simulink model "Regulation_tuning_2024b"  (R2024b)
settings: Solver=FixedStepAuto  StartTime=0.0  StopTime=10.0  FixedStep=0.001  RelTol=1e-3
values from neighbouring files (symbols this model uses):
  theta0 = -pi/2    (= -1.57079632679)    [automated_tuning_simulation.m]    (also in regulation_tuning_simulation.m = 0.785398163397; simulation.m = 0.785398163397; tuning_simulation.m = 0.785398163397)
  x0 = S.traj.xy(1,1)    [automated_tuning_simulation.m]    (also in regulation_tuning_simulation.m = -0.8; simulation.m; tuning_simulation.m)
  x_box = 850    [parking_box.mat]    (also in regulation_tuning_simulation.m = 0; replay_q_timeseries_on_maze_pacman.m; replay_q_timeseries_on_maze_pacman_real.m; simulation.m)
  y0 = S.traj.xy(1,2)    [automated_tuning_simulation.m]    (also in regulation_tuning_simulation.m = 0.5; simulation.m; tuning_simulation.m)
  y_box = 880    [parking_box.mat]    (also in regulation_tuning_simulation.m = 0; replay_q_timeseries_on_maze_pacman.m; replay_q_timeseries_on_maze_pacman_real.m; simulation.m)
undefined symbols (not defined in the file or in its folder): kd, kv, kw
settings Model: Creator=david  LastModifiedBy=emica
settings DataIOCC: ReturnWorkspaceOutputs=off

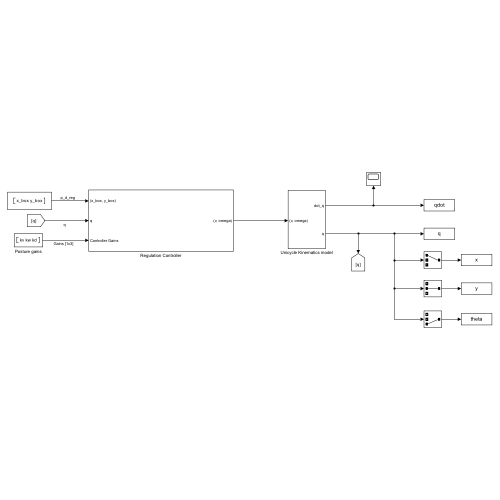
[thumbnail: Simulink's stored preview of the top-level diagram]
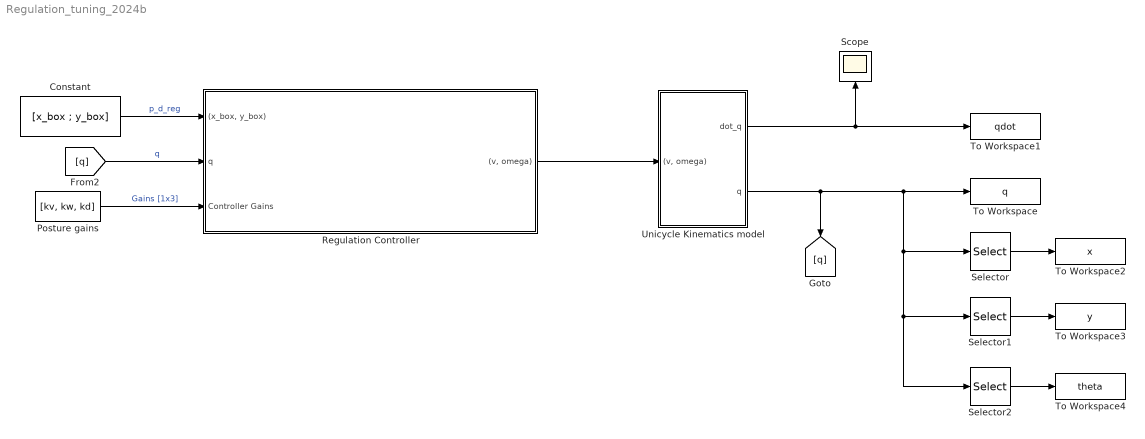
== system Regulation_tuning_2024b ==
  Constant : Constant  Value=[x_box ; y_box]
  Posture gains : Constant  Value=[kv, kw, kd]
  Regulation Controller : Subsystem
  Scope : Scope
  Selector : Selector  InputPortWidth=3  IndexOptions=Index vector (dialog)  Indices=[1]  OutputSizes=1
  Selector1 : Selector  InputPortWidth=3  IndexOptions=Index vector (dialog)  Indices=[2]  OutputSizes=1
  Selector2 : Selector  InputPortWidth=3  IndexOptions=Index vector (dialog)  Indices=[3]  OutputSizes=1
  To Workspace : ToWorkspace  VariableName=q  SaveFormat=Timeseries  SampleTime=-1
  To Workspace1 : ToWorkspace  VariableName=qdot  SaveFormat=Timeseries  SampleTime=-1
  To Workspace2 : ToWorkspace  VariableName=x  SaveFormat=Timeseries  SampleTime=-1
  To Workspace3 : ToWorkspace  VariableName=y  SaveFormat=Timeseries  SampleTime=-1
  To Workspace4 : ToWorkspace  VariableName=theta  SaveFormat=Timeseries  SampleTime=-1
  Unicycle Kinematics model : Subsystem
  wires:
  Regulation Controller/1("(v, omega)") -> Unicycle Kinematics model/1("(v, omega)")
  Constant/1 -> Regulation Controller/1("(x_box, y_box)")  "p_d_reg"
  Unicycle Kinematics model/1(dot_q) -> To Workspace1/1, Scope/1
  [q] -> Regulation Controller/2(q)  "q"
  Posture gains/1 -> Regulation Controller/3(Controller Gains)  "Gains [1x3]"
  Selector/1 -> To Workspace2/1
  Selector1/1 -> To Workspace3/1
  Selector2/1 -> To Workspace4/1
  Unicycle Kinematics model/2(q) -> Selector2/1, Selector1/1, Selector/1, To Workspace/1, [q]

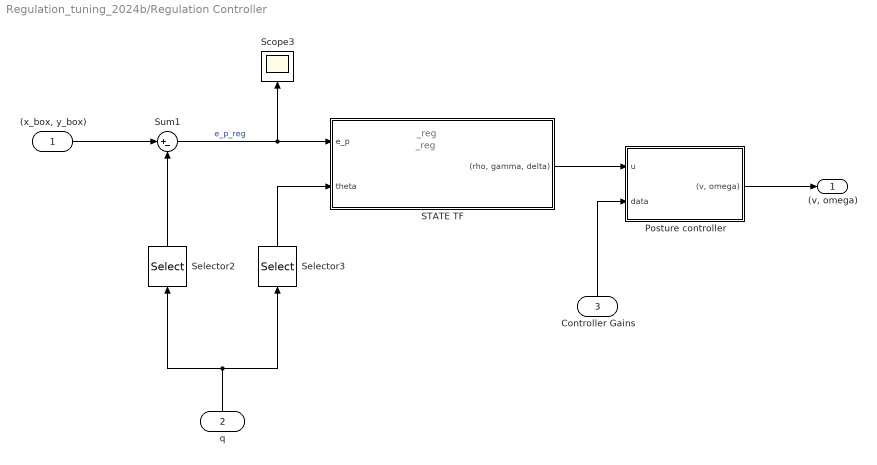
== system Regulation_tuning_2024b/Regulation Controller ==
  note: _reg
  note: _reg
  "(x_box, y_box)" : Inport
  q : Inport  Port=2
  Controller Gains : Inport  Port=3
  Posture controller : Subsystem
  "STATE TF " : Subsystem
  Scope3 : Scope
  Selector2 : Selector  InputPortWidth=3  IndexOptions=Index vector (dialog)  Indices=[1 2]  OutputSizes=1
  Selector3 : Selector  InputPortWidth=3  IndexOptions=Index vector (dialog)  Indices=[3]  OutputSizes=1
  Sum1 : Sum  Inputs=|+-
  "(v, omega)" : Outport
  wires:
  Selector2/1 -> Sum1/2
  Sum1/1 -> "STATE TF "/1(e_p), Scope3/1  "e_p_reg"
  Selector3/1 -> "STATE TF "/2(theta)
  "STATE TF "/1("(rho, gamma, delta)") -> Posture controller/1(u)
  q/1 -> Selector3/1, Selector2/1
  Controller Gains/1 -> Posture controller/2(data)
  Posture controller/1("(v, omega)") -> "(v, omega)"/1
  "(x_box, y_box)"/1 -> Sum1/1

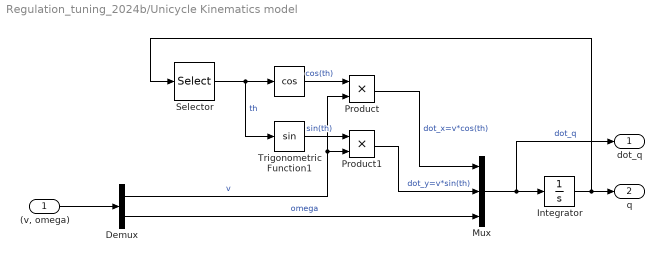
== system Regulation_tuning_2024b/Unicycle Kinematics model ==
  "(v, omega)" : Inport
  " " : Trigonometry  Operator=cos
  Demux : Demux  Outputs=2
  Integrator : Integrator  InitialCondition=[x0; y0; theta0]
  Mux : Mux  Inputs=3
  Product : Product
  Product1 : Product
  Selector : Selector  InputPortWidth=3  IndexOptions=Index vector (dialog)  Indices=[3]  OutputSizes=1
  Trigonometric Function1 : Trigonometry
  dot_q : Outport
  q : Outport  Port=2
  wires:
  Integrator/1 -> Selector/1, q/1
  "(v, omega)"/1 -> Demux/1
  Mux/1 -> Integrator/1, dot_q/1  "dot_q"
  Demux/2 -> Mux/3  "omega"
  Selector/1 -> Trigonometric Function1/1, " "/1  "th"
  " "/1 -> Product/1  "cos(th)"
  Trigonometric Function1/1 -> Product1/1  "sin(th)"
  Demux/1 -> Product1/2, Product/2  "v"
  Product1/1 -> Mux/2  "dot_y=v*sin(th)"
  Product/1 -> Mux/1  "dot_x=v*cos(th)"

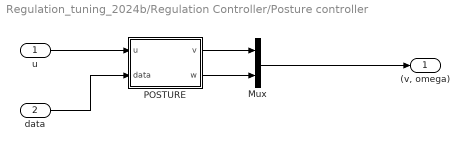
== system Regulation_tuning_2024b/Regulation Controller/Posture controller ==
  u : Inport
  data : Inport  Port=2
  Mux : Mux  Inputs=2
  POSTURE : MATLAB Function  TreatAsAtomicUnit=on
  "(v, omega)" : Outport
  wires:
  POSTURE/2(w) -> Mux/2
  u/1 -> POSTURE/1(u)
  Mux/1 -> "(v, omega)"/1
  data/1 -> POSTURE/2(data)
  POSTURE/1(v) -> Mux/1

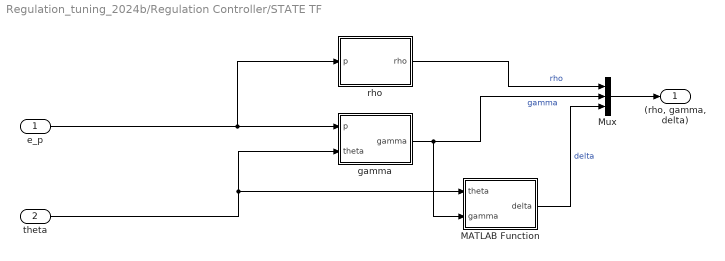
== system Regulation_tuning_2024b/Regulation Controller/STATE TF  ==
  e_p : Inport
  theta : Inport  Port=2
  MATLAB Function : MATLAB Function  TreatAsAtomicUnit=on
  Mux : Mux  Inputs=3
  gamma : MATLAB Function  TreatAsAtomicUnit=on
  rho : MATLAB Function  TreatAsAtomicUnit=on
  "(rho, gamma, delta)" : Outport
  wires:
  gamma/1(gamma) -> Mux/2, MATLAB Function/2(gamma)  "gamma"
  rho/1(rho) -> Mux/1  "rho"
  MATLAB Function/1(delta) -> Mux/3  "delta"
  Mux/1 -> "(rho, gamma, delta)"/1
  e_p/1 -> rho/1(p), gamma/1(p)
  theta/1 -> MATLAB Function/1(theta), gamma/2(theta)

== matlab function Regulation_tuning_2024b/Regulation Controller/Posture controller/POSTURE ==
  data: v output; u input; w output; data input
function [v,w]= fcn(u, data)

K1 = data(1);
K2 = data(2);
K3 = data(3);

rho = u(1);
gamma = u(2);
delta = u(3);


v = K1 * rho * cos(gamma);

if abs(gamma) < 1e-6
    s = 1;                 % sin(gamma)/gamma -> 1
else
    s = sin(gamma)/gamma;
end
w = K2*gamma + K1*(s*cos(gamma))*(gamma + K3*delta);

== matlab function Regulation_tuning_2024b/Regulation Controller/STATE TF /gamma ==
  data: p input; gamma output; theta input
function gamma = fcn(p, theta)

e_x = -p(1);
e_y = -p(2);

gamma = atan2(e_y,e_x) + pi - theta;

end

== matlab function Regulation_tuning_2024b/Regulation Controller/STATE TF /rho ==
  data: rho output; p input
function rho = fcn(p)
e_x = -p(1);
e_y = -p(2);
rho = sqrt(e_x^2 + e_y^2);
end

== matlab function Regulation_tuning_2024b/Regulation Controller/STATE TF /MATLAB Function ==
  data: theta input; delta output; gamma input
function delta = fcn(theta, gamma)



delta = theta + gamma;
end
